simulink model "speed_control"  (R2022b)
settings: Solver=FixedStepAuto  StartTime=0.0  StopTime=4  FixedStep=0.0001  MinStep=0.001  RelTol=1e-3
libraries: slpidlib x2
settings Model: Creator=mique  LastModifiedBy=mique

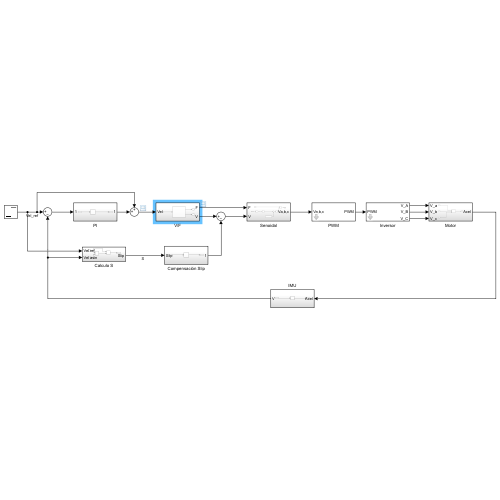
[thumbnail: Simulink's stored preview of the top-level diagram]
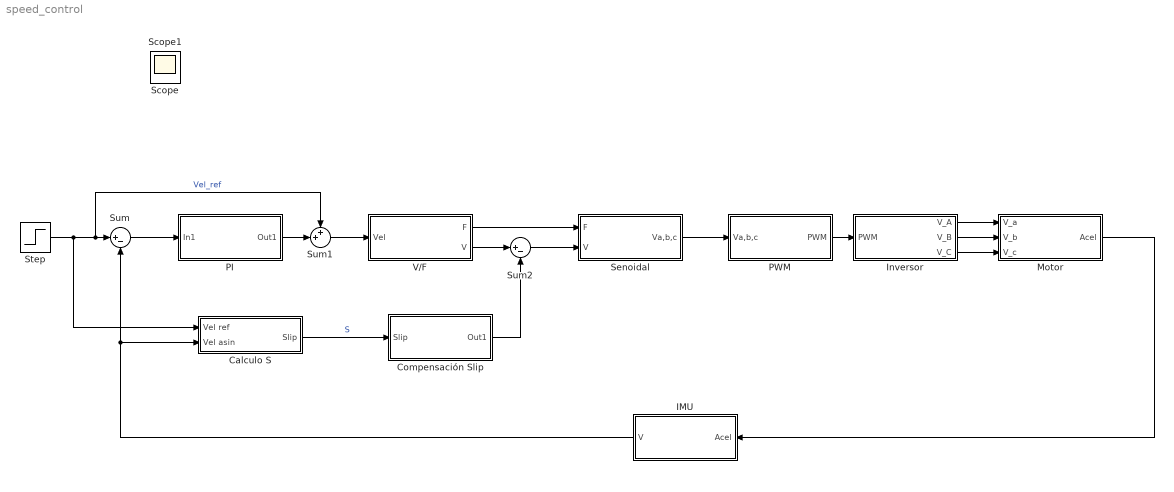
== system speed_control ==
  Calculo S : Subsystem
  Compensación Slip : Subsystem
  IMU : Subsystem
  Inversor : Subsystem  mask{Vmax=220}
      mask prompts: Vmax "Voltaje Maximo"
  Motor : Subsystem
  PI : Subsystem
  PWM : Subsystem  mask{Vmax=220}
      mask prompts: Vmax "Voltaje Maximo"
  Senoidal : Subsystem
  Step : Step  Time=2  Before=1  After=2  SampleTime=0
  Sum : Sum  Inputs=|+-
  Sum1 : Sum  Inputs=++|
  Sum2 : Sum  Inputs=|+-
  V/F : Subsystem
  Scope : Scope
  Scope1 : Scope
  wires:
  Sum1/1 -> V/F/1(Vel)
  PI/1(Out1) -> Sum1/2
  Step/1 -> Calculo S/1(Vel ref), Sum1/1, Sum/1  "Vel_ref"
  Sum/1 -> PI/1(In1)
  Motor/1(Acel) -> IMU/1(Acel)
  IMU/1(V) -> Sum/2, Calculo S/2(Vel asin)
  Senoidal/1(Va,b,c) -> PWM/1(Va,b,c)
  PWM/1(PWM) -> Inversor/1(PWM)
  Inversor/1(V_A) -> Motor/1(V_a)
  Inversor/2(V_B) -> Motor/2(V_b)
  Inversor/3(V_C) -> Motor/3(V_c)
  Calculo S/1(Slip) -> Compensación Slip/1(Slip)  "S"
  V/F/2(V) -> Sum2/1
  Compensación Slip/1(Out1) -> Sum2/2
  Sum2/1 -> Senoidal/2(V)
  V/F/1(F) -> Senoidal/1(F)

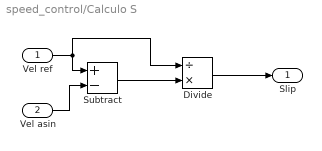
== system speed_control/Calculo S ==
  Vel ref : Inport
  Vel asin : Inport  Port=2
  Divide : Product  Inputs=/*
  Subtract : Sum  Inputs=+-
  Slip : Outport
  wires:
  Vel ref/1 -> Subtract/1, Divide/1
  Vel asin/1 -> Subtract/2
  Divide/1 -> Slip/1
  Subtract/1 -> Divide/2

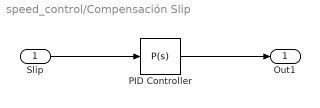
== system speed_control/Compensación Slip ==
  Slip : Inport
  PID Controller : slpidlib/PID Controller  Controller=P  Form=Parallel  TimeDomain=Continuous-time  UseExternalTs=off  SampleTime=-1  IntegratorMethod=Forward Euler  FilterMethod=Forward Euler  ControllerParametersSource=internal  P=1  I=1  UseKiTs=off  D=0  N=100  UseFilter=on  TunerSelectOption=Transfer Function Based (PID Tuner App)  InitialConditionSource=internal  InitialConditionForIntegrator=0  InitialConditionForFilter=0  DifferentiatorICPrevScaledInput=0  ExternalReset=none  TrackingMode=off  Kt=1  LimitOutput=off  SatLimitsSource=internal  UpperSaturationLimit=inf  LowerSaturationLimit=-inf  LinearizeAsGain=on  AntiWindupMode=none  Kb=1  LimitIntegrator=off  UpperIntegratorSaturationLimit=inf  LowerIntegratorSaturationLimit=-inf  POutMin=[]  POutMax=[]  IOutMin=[]  IOutMax=[]  DOutMin=[]  DOutMax=[]  NOutMin=[]  NOutMax=[]  SumOutMin=[]  SumOutMax=[]  SaturationOutMin=[]  SaturationOutMax=[]  PParamMin=[]  PParamMax=[]  IParamMin=[]  IParamMax=[]  DParamMin=[]  DParamMax=[]  NParamMin=[]  NParamMax=[]  KbParamMin=[]  KbParamMax=[]  KtParamMin=[]  KtParamMax=[]  KbOutMin=[]  KbOutMax=[]  KtOutMin=[]  KtOutMax=[]  IntegratorOutMin=[]  IntegratorOutMax=[]  FilterOutMin=[]  FilterOutMax=[]  SumI1OutMin=[]  SumI1OutMax=[]  SumI2OutMin=[]  SumI2OutMax=[]  SumI3OutMin=[]  SumI3OutMax=[]  SumI4OutMin=[]  SumI4OutMax=[]  SumDOutMin=[]  SumDOutMax=[]  DifferentiatorOutMin=[]  DifferentiatorOutMax=[]  FilterDiffOutCoefMin=[]  FilterDiffOutCoefMax=[]  ReciprocalOutMin=[]  ReciprocalOutMax=[]  SumDenOutMin=[]  SumDenOutMax=[]  SumNumOutMin=[]  SumNumOutMax=[]  DivideOutMin=[]  DivideOutMax=[]  UdiffTsProdOutMin=[]  UdiffTsProdOutMax=[]  NTsProdOutMin=[]  NTsProdOutMax=[]  UintegralTsProdOutMin=[]  UintegralTsProdOutMax=[]  UngainTsProdOutMin=[]  UngainTsProdOutMax=[]  ClampingZeroOutDataTypeStr=Inherit: Inherit via back propagation  ClampingZeroOutMin=[]  ClampingZeroOutMax=[]  FilterDenConstantOutDataTypeStr=Inherit: Inherit via back propagation  FilterDenConstantOutMin=[]  FilterDenConstantOutMax=[]  PCopyOutDataTypeStr=Inherit: Inherit via back propagation  PCopyOutMin=[]  PCopyOutMax=[]  NCopyOutDataTypeStr=Inherit: Inherit via back propagation  NCopyOutMin=[]  NCopyOutMax=[]  IntegratorContinuousStateAttributes=''  IntegratorStateMustResolveToSignalObject=off  IntegratorRTWStateStorageClass=Auto  FilterContinuousStateAttributes=''  FilterStateMustResolveToSignalObject=off  FilterRTWStateStorageClass=Auto  ParallelPVariant=InternalParameters  IdealPVariant=Disabled  IVariant=Disabled  DVariant=Disabled  IntegratorVariant=Disabled  SatVariant=Disabled  AWVariant=Disabled  PCopyVariant=Disabled  TRVariant=Disabled  FdbkBlocksVariant=Forward  IdealPFdbkVariant=Disabled  SatFdbkVariant=Disabled  DerivativeFilterVariant=Disabled  NVariant=Disabled  NCopyVariant=Disabled_SignalSpec  FilterICVariant=Disabled  IntegratorICVariant=Disabled  ExternalResetVariant=Disabled  TRSumVariant=Passthrough  SumFdbkVariant=Disabled  SumVariant=Passthrough_P  TsampFilterVariant=InternalTs  TsampNgainVariant=Passthrough  TsampIntegralVariant=Disabled_SignalSpec  ExternalSaturationOutDataTypeStr=Inherit: Same as second input
  Out1 : Outport
  wires:
  Slip/1 -> PID Controller/1
  PID Controller/1 -> Out1/1

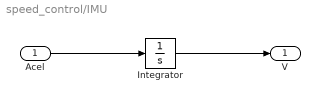
== system speed_control/IMU ==
  Acel : Inport
  Integrator : Integrator  InitialCondition=1
  V : Outport
  wires:
  Acel/1 -> Integrator/1
  Integrator/1 -> V/1

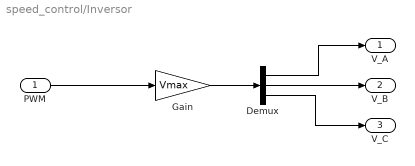
== system speed_control/Inversor ==
  PWM : Inport
  Demux : Demux  Outputs=3
  Gain : Gain  Gain=Vmax
  V_A : Outport
  V_B : Outport  Port=2
  V_C : Outport  Port=3
  wires:
  PWM/1 -> Gain/1
  Demux/1 -> V_A/1
  Gain/1 -> Demux/1
  Demux/2 -> V_B/1
  Demux/3 -> V_C/1

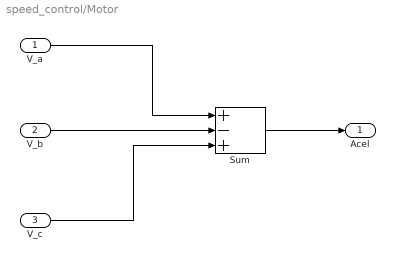
== system speed_control/Motor ==
  V_a : Inport
  V_b : Inport  Port=2
  V_c : Inport  Port=3
  Sum : Sum  Inputs=+-+
  Acel : Outport
  wires:
  V_a/1 -> Sum/1
  V_b/1 -> Sum/2
  Sum/1 -> Acel/1
  V_c/1 -> Sum/3

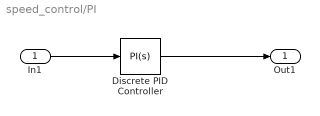
== system speed_control/PI ==
  In1 : Inport
  Discrete PID Controller : slpidlib/PID Controller  Controller=PI  Form=Parallel  TimeDomain=Continuous-time  UseExternalTs=off  SampleTime=-1  IntegratorMethod=Forward Euler  FilterMethod=Forward Euler  ControllerParametersSource=internal  P=1  I=1  UseKiTs=off  D=0  N=100  UseFilter=on  TunerSelectOption=Transfer Function Based (PID Tuner App)  InitialConditionSource=internal  InitialConditionForIntegrator=0  InitialConditionForFilter=0  DifferentiatorICPrevScaledInput=0  ExternalReset=none  TrackingMode=off  Kt=1  LimitOutput=off  SatLimitsSource=internal  UpperSaturationLimit=inf  LowerSaturationLimit=-inf  LinearizeAsGain=off  AntiWindupMode=none  Kb=1  LimitIntegrator=off  UpperIntegratorSaturationLimit=inf  LowerIntegratorSaturationLimit=-inf  POutMin=[]  POutMax=[]  IOutMin=[]  IOutMax=[]  DOutMin=[]  DOutMax=[]  NOutMin=[]  NOutMax=[]  SumOutMin=[]  SumOutMax=[]  SaturationOutMin=[]  SaturationOutMax=[]  PParamMin=[]  PParamMax=[]  IParamMin=[]  IParamMax=[]  DParamMin=[]  DParamMax=[]  NParamMin=[]  NParamMax=[]  KbParamMin=[]  KbParamMax=[]  KtParamMin=[]  KtParamMax=[]  KbOutMin=[]  KbOutMax=[]  KtOutMin=[]  KtOutMax=[]  IntegratorOutMin=[]  IntegratorOutMax=[]  FilterOutMin=[]  FilterOutMax=[]  SumI1OutMin=[]  SumI1OutMax=[]  SumI2OutMin=[]  SumI2OutMax=[]  SumI3OutMin=[]  SumI3OutMax=[]  SumI4OutMin=[]  SumI4OutMax=[]  SumDOutMin=[]  SumDOutMax=[]  DifferentiatorOutMin=[]  DifferentiatorOutMax=[]  FilterDiffOutCoefMin=[]  FilterDiffOutCoefMax=[]  ReciprocalOutMin=[]  ReciprocalOutMax=[]  SumDenOutMin=[]  SumDenOutMax=[]  SumNumOutMin=[]  SumNumOutMax=[]  DivideOutMin=[]  DivideOutMax=[]  UdiffTsProdOutMin=[]  UdiffTsProdOutMax=[]  NTsProdOutMin=[]  NTsProdOutMax=[]  UintegralTsProdOutMin=[]  UintegralTsProdOutMax=[]  UngainTsProdOutMin=[]  UngainTsProdOutMax=[]  ClampingZeroOutDataTypeStr=Inherit: Inherit via back propagation  ClampingZeroOutMin=[]  ClampingZeroOutMax=[]  FilterDenConstantOutDataTypeStr=Inherit: Inherit via back propagation  FilterDenConstantOutMin=[]  FilterDenConstantOutMax=[]  PCopyOutDataTypeStr=Inherit: Inherit via back propagation  PCopyOutMin=[]  PCopyOutMax=[]  NCopyOutDataTypeStr=Inherit: Inherit via back propagation  NCopyOutMin=[]  NCopyOutMax=[]  IntegratorContinuousStateAttributes=''  IntegratorStateMustResolveToSignalObject=off  IntegratorRTWStateStorageClass=Auto  FilterContinuousStateAttributes=''  FilterStateMustResolveToSignalObject=off  FilterRTWStateStorageClass=Auto  ParallelPVariant=InternalParameters  IdealPVariant=Disabled  IVariant=InternalParameters  DVariant=Disabled  IntegratorVariant=Continuous  SatVariant=Disabled  AWVariant=Passthrough  PCopyVariant=Disabled  TRVariant=Disabled  FdbkBlocksVariant=Forward  IdealPFdbkVariant=Disabled  SatFdbkVariant=Disabled  DerivativeFilterVariant=Disabled  NVariant=Disabled  NCopyVariant=Disabled_SignalSpec  FilterICVariant=Disabled  IntegratorICVariant=InternalICs  ExternalResetVariant=Disabled  TRSumVariant=Passthrough  SumFdbkVariant=Disabled  SumVariant=Sum_PI  TsampFilterVariant=InternalTs  TsampNgainVariant=Passthrough  TsampIntegralVariant=Passthrough  ExternalSaturationOutDataTypeStr=Inherit: Same as second input
      settings: LibrarySourceBlock=simulink/Discrete/Discrete PID Controller
  Out1 : Outport
  wires:
  In1/1 -> Discrete PID Controller/1
  Discrete PID Controller/1 -> Out1/1

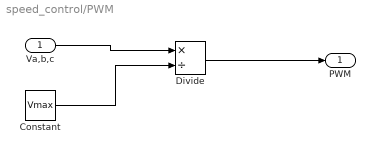
== system speed_control/PWM ==
  Va,b,c : Inport
  Constant : Constant  Value=Vmax
  Divide : Product  Inputs=*/
  PWM : Outport
  wires:
  Va,b,c/1 -> Divide/1
  Constant/1 -> Divide/2
  Divide/1 -> PWM/1

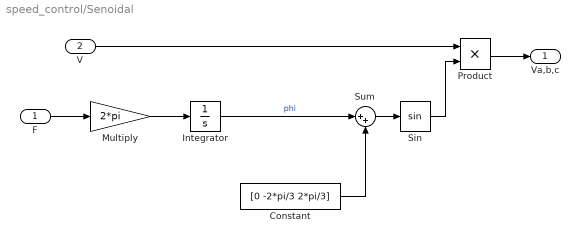
== system speed_control/Senoidal ==
  F : Inport
  V : Inport  Port=2
  Constant : Constant  Value=[0 -2*pi/3 2*pi/3]
  Integrator : Integrator  WrapState=on  WrappedStateUpperValue=2*pi  WrappedStateLowerValue=-2*pi
  Multiply : Gain  Gain=2*pi
  Product : Product
  Sin : Trigonometry
  Sum : Sum  Inputs=|++
  Va,b,c : Outport
  wires:
  Integrator/1 -> Sum/1  "phi"
  Constant/1 -> Sum/2
  Sum/1 -> Sin/1
  V/1 -> Product/1
  Sin/1 -> Product/2
  Product/1 -> Va,b,c/1
  F/1 -> Multiply/1
  Multiply/1 -> Integrator/1

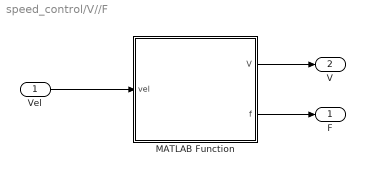
== system speed_control/V//F ==
  Vel : Inport
  MATLAB Function : MATLAB Function  TreatAsAtomicUnit=on
  F : Outport
  V : Outport  Port=2
  wires:
  Vel/1 -> MATLAB Function/1(vel)
  MATLAB Function/1(V) -> V/1
  MATLAB Function/2(f) -> F/1

== matlab function speed_control/V//F/MATLAB Function ==
  data: vel input; V output; f output
function [V,f]= v_f(vel)

pasoPolar=0.114;

f=vel/(2*pasoPolar);

%Comprobar valores
f_corte_inf=6;
V_min=40;
V_max=220;
f_corte_sup=f_corte_inf*V_max/V_min;

if(f<f_corte_inf)
    V=V_min;
    disp('aqui')
elseif(f<f_corte_sup)
    V=V_min/f_corte_inf*f;
    disp('lineal')
else
    V=V_max;
    disp('fuera')
end
